simulink model "Generator_Beam"  (R2022b)
settings: Solver=VariableStepAuto  StartTime=0.0  StopTime=10.0  RelTol=1e-3
model workspace (MAT data in the model file):
  QL = Simulink.Parameter
  QL.Value = 960000
  QL.DataType = 'auto'
  QL.Complexity = 'real'
  QL.Dimensions = [1 1]
  RL = Simulink.Parameter
  RL.Value = Simulink.data.Expression
  RL.Value.ExpressionString = "RQ*QL"
  RL.DataType = 'auto'
  RL.Complexity = 'real'
  RL.Dimensions = -1
  RQ = Simulink.Parameter
  RQ.Value = 310
  RQ.DataType = 'auto'
  RQ.Complexity = 'real'
  RQ.Dimensions = [1 1]
  Ts = Simulink.Parameter
  Ts.Value = 1e-10
  Ts.DataType = 'auto'
  Ts.Complexity = 'real'
  Ts.Dimensions = [1 1]
  f0 = Simulink.Parameter
  f0.Value = 648000000
  f0.DataType = 'auto'
  f0.Complexity = 'real'
  f0.Dimensions = [1 1]
  w_hbw = Simulink.Parameter
  w_hbw.Value = Simulink.data.Expression
  w_hbw.Value.ExpressionString = "pi*f0/QL"
  w_hbw.DataType = 'auto'
  w_hbw.Complexity = 'real'
  w_hbw.Dimensions = -1
settings Model: Creator=mliu  LastModifiedBy=mliu

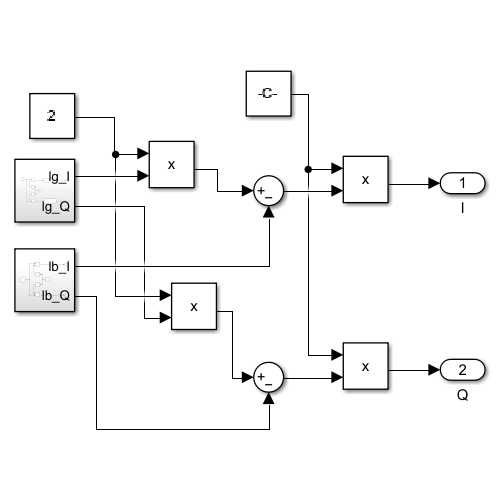
[thumbnail: Simulink's stored preview of the top-level diagram]
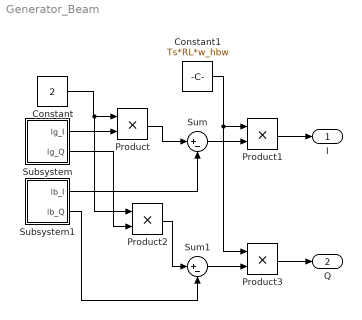
== system Generator_Beam ==
  Constant : Constant  Value=2
  Constant1 : Constant  Value=Ts*RL*w_hbw
  Product{,1..3} (4 alike) : Product
  Subsystem : Subsystem
  Subsystem1 : Subsystem
  Sum : Sum  Inputs=|+-
  Sum1 : Sum  Inputs=|+-
  I : Outport
  Q : Outport  Port=2
  wires:
  Subsystem/1(lg_I) -> Product/2
  Constant/1 -> Product2/1, Product/1
  Product/1 -> Sum/1
  Subsystem1/1(lb_I) -> Sum/2
  Sum/1 -> Product1/2
  Constant1/1 -> Product3/1, Product1/1
  Product1/1 -> I/1
  Subsystem/2(lg_Q) -> Product2/2
  Product2/1 -> Sum1/1
  Subsystem1/2(lb_Q) -> Sum1/2
  Sum1/1 -> Product3/2
  Product3/1 -> Q/1

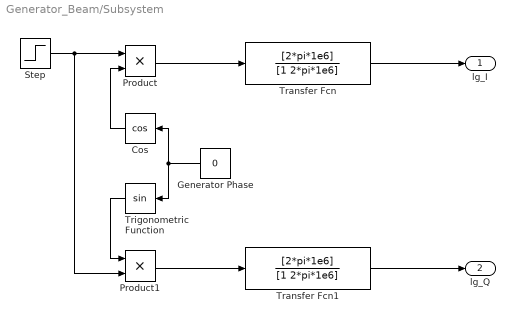
== system Generator_Beam/Subsystem ==
  Cos : Trigonometry  Operator=cos
  Generator Phase : Constant  Value=0
  Product : Product
  Product1 : Product
  Step : Step  SampleTime=0
  Transfer Fcn : TransferFcn  Numerator=[2*pi*1e6]  Denominator=[1 2*pi*1e6]
  Transfer Fcn1 : TransferFcn  Numerator=[2*pi*1e6]  Denominator=[1 2*pi*1e6]
  Trigonometric Function : Trigonometry
  lg_I : Outport
  lg_Q : Outport  Port=2
  wires:
  Generator Phase/1 -> Trigonometric Function/1, Cos/1
  Transfer Fcn1/1 -> lg_Q/1
  Product1/1 -> Transfer Fcn1/1
  Trigonometric Function/1 -> Product1/1
  Transfer Fcn/1 -> lg_I/1
  Cos/1 -> Product/2
  Product/1 -> Transfer Fcn/1
  Step/1 -> Product1/2, Product/1

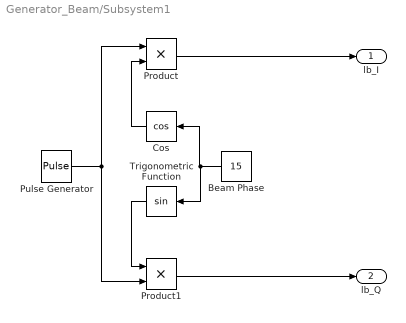
== system Generator_Beam/Subsystem1 ==
  Beam Phase : Constant  Value=15
  Cos : Trigonometry  Operator=cos
  Product : Product
  Product1 : Product
  Pulse Generator : DiscretePulseGenerator  PulseType=Time based  Period=0.04  PulseWidth=5
  Trigonometric Function : Trigonometry
  lb_I : Outport
  lb_Q : Outport  Port=2
  wires:
  Product/1 -> lb_I/1
  Trigonometric Function/1 -> Product1/1
  Pulse Generator/1 -> Product/1, Product1/2
  Beam Phase/1 -> Trigonometric Function/1, Cos/1
  Product1/1 -> lb_Q/1
  Cos/1 -> Product/2
